simulink model "PMSM_PFC_ESO"  (R2023b)
settings: Solver=ode4  StartTime=0.0  StopTime=0.8  FixedStep=5e-6  RelTol=1e-3
settings Model: Creator=Y  LastModifiedBy=Y

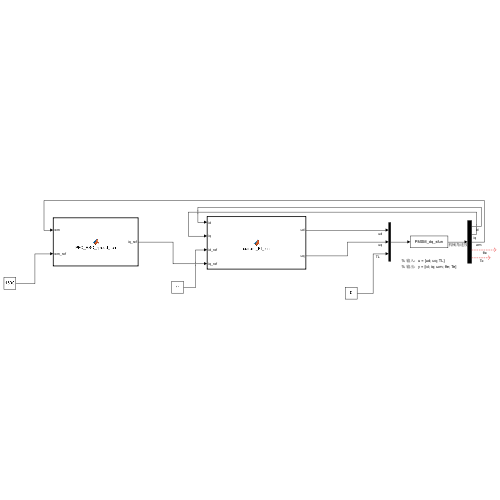
[thumbnail: Simulink's stored preview of the top-level diagram]
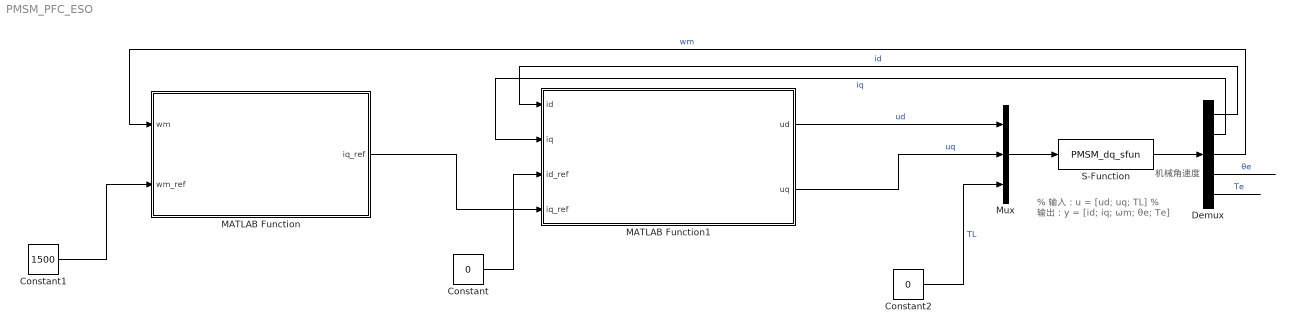
== system PMSM_PFC_ESO ==
  note: 机械角速度
  note: % 输入：u = [ud; uq; TL]
      | % 输出：y = [id; iq; ωm; θe; Te]
  Constant : Constant  Value=0
  Constant1 : Constant  Value=1500
  Constant2 : Constant  Value=0
  Demux : Demux  Outputs=5
  MATLAB Function : MATLAB Function  TreatAsAtomicUnit=on
  MATLAB Function1 : MATLAB Function  TreatAsAtomicUnit=on
  Mux : Mux  Inputs=3
  S-Function : S-Function  FunctionName=PMSM_dq_sfun  SFunctionDeploymentMode=off  EnableBusSupport=off
  wires:
  Mux/1 -> S-Function/1
  S-Function/1 -> Demux/1
  Demux/1 -> MATLAB Function1/1(id)  "id"
  Demux/2 -> MATLAB Function1/2(iq)  "iq"
  Demux/3 -> MATLAB Function/1(wm)  "wm"
  Demux/4 -> ?  "θe"
  Demux/5 -> ?  "Te"
  MATLAB Function1/1(ud) -> Mux/1  "ud"
  MATLAB Function1/2(uq) -> Mux/2  "uq"
  Constant2/1 -> Mux/3  "TL"
  MATLAB Function/1(iq_ref) -> MATLAB Function1/4(iq_ref)
  Constant/1 -> MATLAB Function1/3(id_ref)
  Constant1/1 -> MATLAB Function/2(wm_ref)

== matlab function PMSM_PFC_ESO/MATLAB Function1 ==
  settings: updateMethod=DISCRETE  sampleTime=60e-6
  data: id input; ud output; iq input; id_ref input; iq_ref input; uq output
function [ud, uq] = current_PI_fcn(id, iq, id_ref, iq_ref)
% dq 电流环 PI
% 论文参数：Kp=50, Ki=2500

Kp = 50;  Ki = 2500;
Ts_i = 60e-6;
Udc = 310;  Us_max = Udc / sqrt(3);

persistent int_d int_q
if isempty(int_d)
    int_d = 0; int_q = 0;
end

ed = id_ref - id;
int_d = int_d + Ki * ed * Ts_i;
ud = Kp * ed + int_d;
ud = max(-Us_max, min(Us_max, ud));

eq = iq_ref - iq;
int_q = int_q + Ki * eq * Ts_i;
uq = Kp * eq + int_q;
uq = max(-Us_max, min(Us_max, uq));
end

== matlab function PMSM_PFC_ESO/MATLAB Function ==
  settings: updateMethod=DISCRETE  sampleTime=250e-6
  data: wm input; iq_ref output; wm_ref input
function iq_ref = PFC_ESO_speed_fcn(wm, wm_ref)
% PFC+ESO 速度控制器
% 输入：wm（实际转速 [rad/s]），wm_ref（参考转速 [rad/s]）
% 输出：iq_ref（q轴电流参考 [A]）

% --- 电机参数 ---
Kt = 1.5 * 4 * 0.1167;       % = 0.7002 N·m/A
J  = 1.74e-4;
Bv = 7.403e-5;
Km = Kt / Bv;                % 稳态增益

% --- PFC 参数（论文值）---
Ts = 250e-6;
Tr = 50e-6;
P  = 3;
r  = 1.8;
alpha_m = 0.999;
alpha_r = exp(-Ts / Tr);

% --- ESO 参数 ---
p_eso = 4000;
b0 = Kt / J;                 % ≈ 5414

% --- iq 限幅 ---
iq_max = 10;

% --- persistent 变量 ---
persistent z1 z2 iq_prev
if isempty(z1)
    z1 = 0; z2 = 0; iq_prev = 0;
end

% --- ESO 更新（论文式23，前向欧拉 + 子步积分）---
% 稳定性要求 h_sub * p_eso < 1，Ts*p_eso = 1.0 恰好在边界
% 因此用子步积分保证稳定
N_eso = ceil(p_eso * Ts / 0.3);   % ≈ 4 子步
h_eso = Ts / N_eso;
for n_eso = 1:N_eso
    err_eso = z1 - wm;
    dz1 = z2 - 2*p_eso*err_eso + b0*iq_prev;
    dz2 = -p_eso^2 * err_eso;
    z1 = z1 + h_eso * dz1;
    z2 = z2 + h_eso * dz2;
end

% --- PFC 控制律（论文式19）---
Wo = zeros(P, 1);
Wb = zeros(P, 1);
Wr = zeros(P, 1);
for i = 1:P
    Wo(i) = alpha_m^i * wm;
    Wb(i) = Km * (1 - alpha_m^i);
    Wr(i) = wm_ref - alpha_r^i * (wm_ref - wm);
end

iq_pfc = (Wb' * (Wr - Wo)) / (Wb' * Wb + r^2);

% --- ESO 前馈补偿（论文式24）---
iq_ref = iq_pfc - z2 / b0;

% --- 限幅 ---
if iq_ref > iq_max
    iq_ref = iq_max;
elseif iq_ref < -iq_max
    iq_ref = -iq_max;
end

iq_prev = iq_ref;
end
